simulink model "test_lift"  (R2021b)
settings: Solver=VariableStepAuto  StartTime=0.0  StopTime=100  MaxStep=1e-3  RelTol=1e-3
values from neighbouring files (symbols this model uses):
  g = 9.806    [plot_bode_diagram.m]    (also in test_LiftDynamicsEquation.m; test_discretization.m)
  num_floors = 20    [test_LiftDynamicsEquation.m]    (also in test_discretization.m)
  Ts = 1e-3    (= 0.001)    [test_LiftDynamicsEquation.m]    (also in test_discretization.m; test_motion_law.m = 0.01)
libraries: LumpedParameterLiftModels x3, cstblocks x2
settings Model: Creator=manue  LastModifiedBy=manue

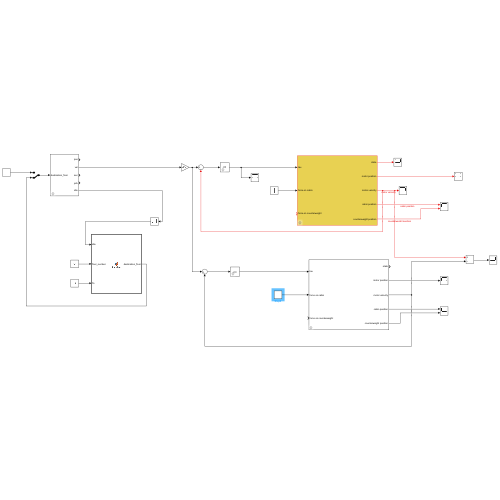
[thumbnail: Simulink's stored preview of the top-level diagram]
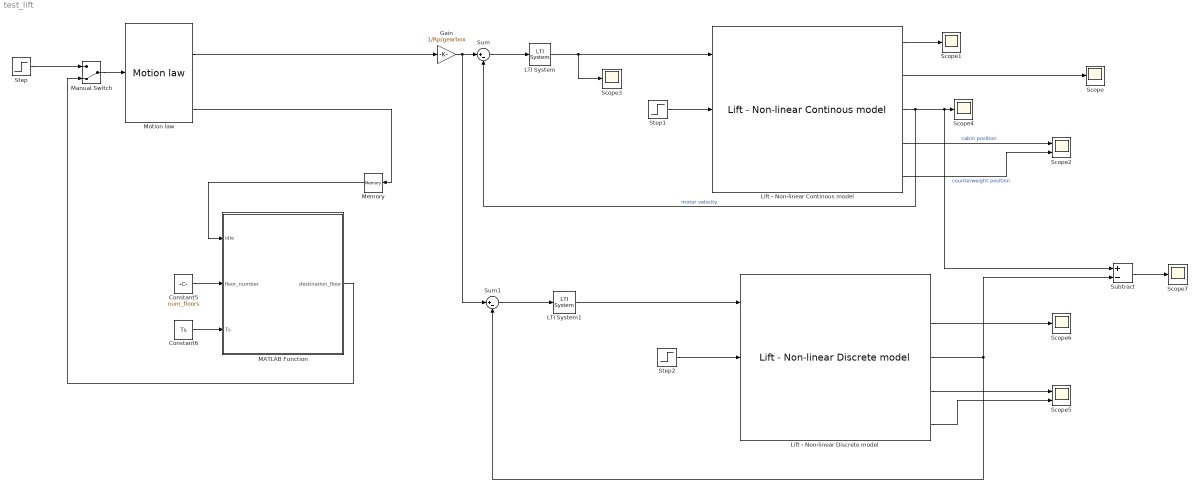
== system test_lift ==
  Constant5 : Constant  Value=num_floors
  Constant6 : Constant  Value=Ts
  Gain : Gain  Gain=1/Rp/gearbox
  LTI System : cstblocks/LTI System  sys=ctrl  IC=[]
  LTI System1 : cstblocks/LTI System  sys=ctrl  IC=[]
  Lift - Non-linear Continous model : LumpedParameterLiftModels/Lift - Non-linear Continous model  Jp=Jp  Jm=Jm  Mc=Mc  Mw=Mw  LinearStiffness=LinearStiffness  LinearDamping=LinearDamping  Rp=Rp  mu=mu  BuildingHeight=BuildingHeight  MotorViscousFriction=MotorViscousFriction  g=g  gearbox=gearbox  min_length=min_length  x9_init=0
  Lift - Non-linear Discrete model : LumpedParameterLiftModels/Lift - Non-linear Discrete model  Jp=Jp  Jm=Jm  Mc=Mc  Mw=Mw  LinearStiffness=LinearStiffness  LinearDamping=LinearDamping  Rp=Rp  mu=mu  BuildingHeight=BuildingHeight  MotorViscousFriction=MotorViscousFriction  g=g  gearbox=gearbox  min_length=min_length  x9_init=0  Ts=Ts
  MATLAB Function : MATLAB Function  TreatAsAtomicUnit=on  SystemSampleTime=Ts
  Manual Switch : ManualSwitch  CurrentSetting=0
  Memory : Memory
  Motion law : LumpedParameterLiftModels/Motion law  MaxVel=MaxVel  MaxAcc=MaxAcc  MaxJerk=MaxJerk  Ts=Ts  floor_height=floor_height
  Scope{,1,3..4,6..7} (6 alike) : Scope
  Scope2 : Scope  NumInputPorts=2
  Scope5 : Scope  NumInputPorts=2
  Step : Step  Time=10  After=15  SampleTime=0
  Step1 : Step  Time=20  After=0  SampleTime=0
  Step2 : Step  Time=20  After=0  SampleTime=0
  Subtract : Sum  Inputs=+-
  Sum : Sum  Inputs=|+-
  Sum1 : Sum  Inputs=|+-
  wires:
  Lift - Non-linear Continous model/2 -> Scope/1
  Lift - Non-linear Continous model/1 -> Scope1/1
  Lift - Non-linear Continous model/4 -> Scope2/1  "cabin position"
  Lift - Non-linear Continous model/5 -> Scope2/2  "counterweight position"
  Step1/1 -> Lift - Non-linear Continous model/2
  Gain/1 -> Sum1/1, Sum/1
  LTI System/1 -> Lift - Non-linear Continous model/1, Scope3/1
  Sum/1 -> LTI System/1
  Lift - Non-linear Continous model/3 -> Subtract/1, Scope4/1, Sum/2  "motor velocity"
  Memory/1 -> MATLAB Function/1(idle)
  Constant5/1 -> MATLAB Function/2(floor_number)
  Constant6/1 -> MATLAB Function/3(Ts)
  MATLAB Function/1(destination_floor) -> Manual Switch/2
  Motion law/2 -> Gain/1
  Motion law/5 -> Memory/1
  Manual Switch/1 -> Motion law/1
  Step/1 -> Manual Switch/1
  LTI System1/1 -> Lift - Non-linear Discrete model/1
  Sum1/1 -> LTI System1/1
  Lift - Non-linear Discrete model/3 -> Sum1/2, Subtract/2
  Lift - Non-linear Discrete model/4 -> Scope5/1
  Lift - Non-linear Discrete model/5 -> Scope5/2
  Lift - Non-linear Discrete model/2 -> Scope6/1
  Subtract/1 -> Scope7/1
  Step2/1 -> Lift - Non-linear Discrete model/2

== matlab function test_lift/MATLAB Function ==
  data: idle input; destination_floor output; floor_number input; Ts input
function destination_floor = Random(idle,floor_number,Ts)

persistent destination_floor_ state time wait_time;
if isempty(destination_floor_)
    destination_floor_=0;
    state=0;
    time=0;
    wait_time=0;
end

if (state==0 && idle) % wait a random time
    wait_time=25+5*rand();
    time=0;
    state=1;
elseif (state==1 && time>wait_time)
    state=2;
elseif (state==2)
    state=0;
end

time=time+Ts;
if (state==2)
    destination_floor_=randi(floor_number);
end

destination_floor=destination_floor_;
